simulink model "StateSpace"  (R2022a)
settings: Solver=ode113  StartTime=0.0  StopTime=10  MaxStep=1e-3  RelTol=1e-6
undefined symbols (not defined in the file): k
settings Model: Creator=Administrator  LastModifiedBy=Administrator
settings SolverCC: NumberNewtonIterations=100  MaxConsecutiveMinStep=10  SolverJacobianMethodControl=FullAnalytical  DaesscMode=FullDebug  ShapePreserveControl=EnableAll  ZeroCrossAlgorithm=Adaptive  SolverResetMethod=Robust  ODENIntegrationMethod=ode14x

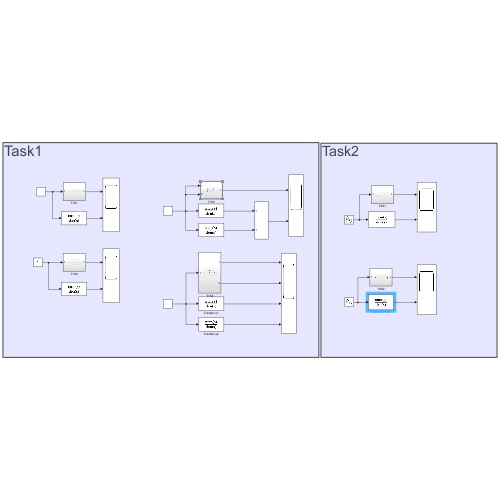
[thumbnail: Simulink's stored preview of the top-level diagram]
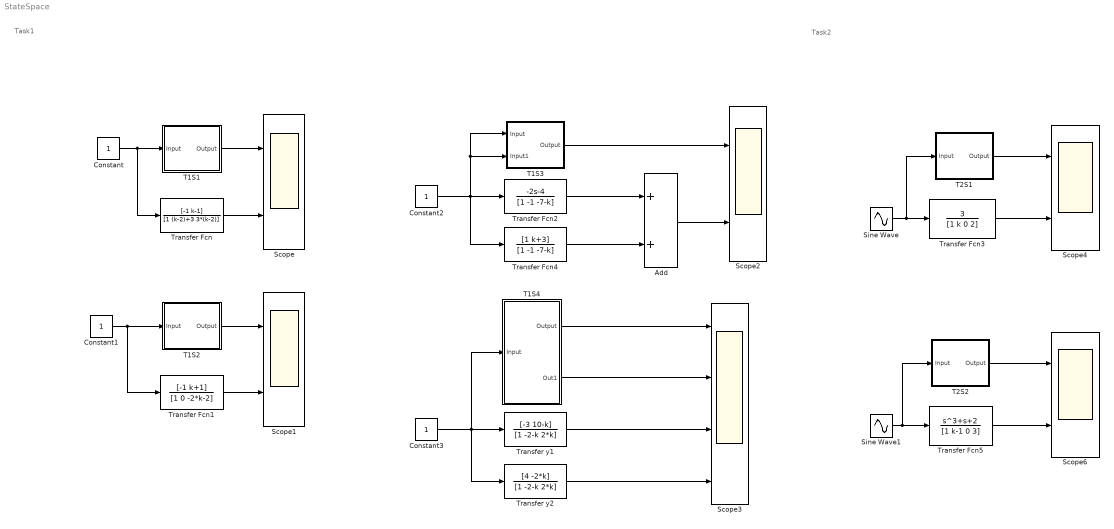
== system StateSpace ==
  note: Task2
  note: Task1
  Add : Sum  RndMeth=Nearest
  Constant{,1..3} (4 alike) : Constant
  Scope{,1..2,4,6} (5 alike) : Scope  NumInputPorts=2
  Scope3 : Scope  NumInputPorts=4
  Sine Wave : Sin  Amplitude=3  Frequency=2  SampleTime=0
  Sine Wave1 : Sin  Amplitude=3  Frequency=2  SampleTime=0
  T1S1 : Subsystem
  T1S2 : Subsystem
  T1S3 : Subsystem
  T1S4 : Subsystem
  T2S1 : Subsystem
  T2S2 : Subsystem
  Transfer Fcn : TransferFcn  Numerator=[-1 k-1]  Denominator=[1 (k-2)+3 3*(k-2)]
  Transfer Fcn1 : TransferFcn  Numerator=[-1 k+1]  Denominator=[1 0 -2*k-2]
  Transfer Fcn2 : TransferFcn  Numerator=[-2 -4]  Denominator=[1 -1 -7-k]
  Transfer Fcn3 : TransferFcn  Numerator=[3]  Denominator=[1 k 0 2]
  Transfer Fcn4 : TransferFcn  Numerator=[1 k+3]  Denominator=[1 -1 -7-k]
  Transfer Fcn5 : TransferFcn  Numerator=[1 0 1 2]  Denominator=[1 k-1 0 3]
  Transfer y1 : TransferFcn  Numerator=[-3 10-k]  Denominator=[1 -2-k 2*k]
  Transfer y2 : TransferFcn  Numerator=[4 -2*k]  Denominator=[1 -2-k 2*k]
  wires:
  Constant/1 -> Transfer Fcn/1, T1S1/1(Input)
  T1S1/1(Output) -> Scope/1
  Transfer Fcn/1 -> Scope/2
  Constant1/1 -> Transfer Fcn1/1, T1S2/1(Input)
  Transfer Fcn1/1 -> Scope1/2
  T1S2/1(Output) -> Scope1/1
  T1S3/1(Output) -> Scope2/1
  Transfer Fcn2/1 -> Add/1
  Constant2/1 -> T1S3/1(Input), T1S3/2(Input1), Transfer Fcn4/1, Transfer Fcn2/1
  Constant3/1 -> T1S4/1(Input), Transfer y2/1, Transfer y1/1
  Transfer y1/1 -> Scope3/3
  T1S4/1(Output) -> Scope3/1
  Add/1 -> Scope2/2
  Transfer Fcn4/1 -> Add/2
  T1S4/2(Out1) -> Scope3/2
  Transfer y2/1 -> Scope3/4
  Sine Wave/1 -> Transfer Fcn3/1, T2S1/1(Input)
  Transfer Fcn3/1 -> Scope4/2
  Sine Wave1/1 -> T2S2/1(Input), Transfer Fcn5/1
  Transfer Fcn5/1 -> Scope6/2
  T2S1/1(Output) -> Scope4/1
  T2S2/1(Output) -> Scope6/1

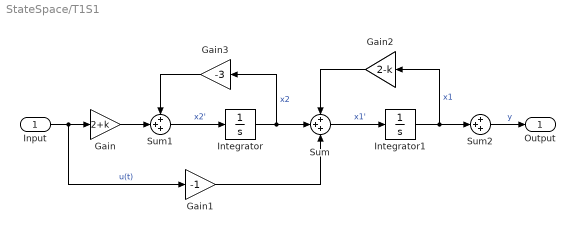
== system StateSpace/T1S1 ==
  Input : Inport
  Gain : Gain  Gain=2+k
  Gain1 : Gain  Gain=-1
  Gain2 : Gain  Gain=2-k
  Gain3 : Gain  Gain=-3
  Integrator : Integrator
  Integrator1 : Integrator
  Sum : Sum  Inputs=+++
  Sum1 : Sum  Inputs=+++
  Sum2 : Sum  Inputs=+++
  Output : Outport
  wires:
  Gain2/1 -> Sum/1
  Sum/1 -> Integrator1/1  "x1'"
  Integrator1/1 -> Sum2/2, Gain2/1  "x1"
  Input/1 -> Gain1/1, Gain/1  "u(t)"
  Gain/1 -> Sum1/2
  Sum1/1 -> Integrator/1  "x2'"
  Integrator/1 -> Gain3/1, Sum/2  "x2"
  Gain1/1 -> Sum/3
  Sum2/1 -> Output/1  "y"
  Gain3/1 -> Sum1/1

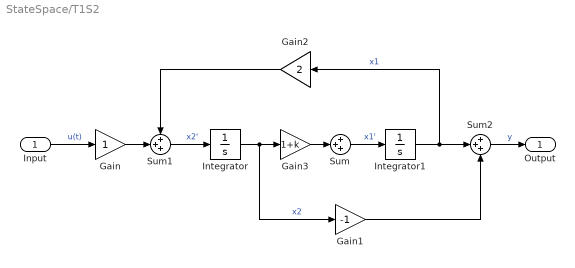
== system StateSpace/T1S2 ==
  Input : Inport
  Gain : Gain
  Gain1 : Gain  Gain=-1
  Gain2 : Gain  Gain=2
  Gain3 : Gain  Gain=1+k
  Integrator : Integrator
  Integrator1 : Integrator
  Sum : Sum  Inputs=+++
  Sum1 : Sum  Inputs=+++
  Sum2 : Sum  Inputs=+++
  Output : Outport
  wires:
  Gain2/1 -> Sum1/1
  Sum/1 -> Integrator1/1  "x1'"
  Integrator1/1 -> Sum2/2, Gain2/1  "x1"
  Input/1 -> Gain/1  "u(t)"
  Gain/1 -> Sum1/2
  Sum1/1 -> Integrator/1  "x2'"
  Integrator/1 -> Gain1/1, Gain3/1  "x2"
  Sum2/1 -> Output/1  "y"
  Gain3/1 -> Sum/2
  Gain1/1 -> Sum2/3

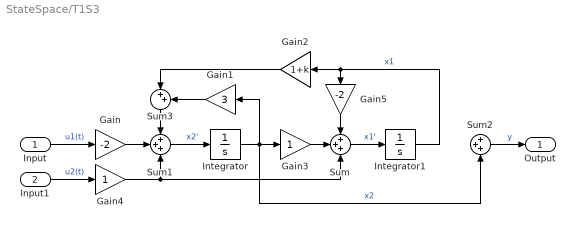
== system StateSpace/T1S3 ==
  Input : Inport
  Input1 : Inport  Port=2
  Gain : Gain  Gain=-2
  Gain1 : Gain  Gain=3
  Gain2 : Gain  Gain=1+k
  Gain3 : Gain
  Gain4 : Gain
  Gain5 : Gain  Gain=-2
  Integrator : Integrator
  Integrator1 : Integrator
  Sum : Sum  Inputs=+++
  Sum1 : Sum  Inputs=+++
  Sum2 : Sum  Inputs=+++
  Sum3 : Sum  Inputs=|++
  Output : Outport
  wires:
  Gain2/1 -> Sum3/1
  Sum/1 -> Integrator1/1  "x1'"
  Integrator1/1 -> Gain2/1, Gain5/1  "x1"
  Input/1 -> Gain/1  "u1(t)"
  Gain/1 -> Sum1/2
  Sum1/1 -> Integrator/1  "x2'"
  Integrator/1 -> Sum2/3, Gain1/1, Gain3/1  "x2"
  Sum2/1 -> Output/1  "y"
  Gain3/1 -> Sum/2
  Input1/1 -> Gain4/1  "u2(t)"
  Gain4/1 -> Sum/3, Sum1/3
  Sum3/1 -> Sum1/1
  Gain1/1 -> Sum3/2
  Gain5/1 -> Sum/1

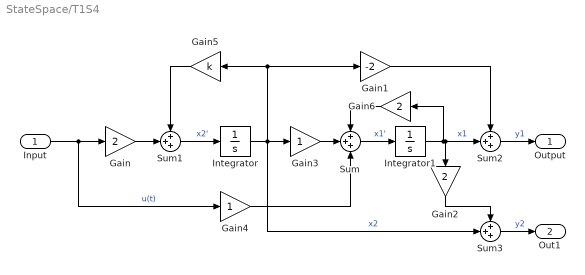
== system StateSpace/T1S4 ==
  Input : Inport
  Gain : Gain  Gain=2
  Gain1 : Gain  Gain=-2
  Gain2 : Gain  Gain=2
  Gain3 : Gain
  Gain4 : Gain
  Gain5 : Gain  Gain=k
  Gain6 : Gain  Gain=2
  Integrator : Integrator
  Integrator1 : Integrator
  Sum{,1..3} (4 alike) : Sum  Inputs=+++
  Output : Outport
  Out1 : Outport  Port=2
  wires:
  Sum/1 -> Integrator1/1  "x1'"
  Integrator1/1 -> Gain6/1, Sum2/2, Gain2/1  "x1"
  Input/1 -> Gain4/1, Gain/1  "u(t)"
  Gain/1 -> Sum1/2
  Sum1/1 -> Integrator/1  "x2'"
  Integrator/1 -> Gain3/1, Gain1/1, Gain5/1, Sum3/2  "x2"
  Sum2/1 -> Output/1  "y1"
  Gain3/1 -> Sum/2
  Sum3/1 -> Out1/1  "y2"
  Gain1/1 -> Sum2/1
  Gain2/1 -> Sum3/1
  Gain4/1 -> Sum/3
  Gain5/1 -> Sum1/1
  Gain6/1 -> Sum/1

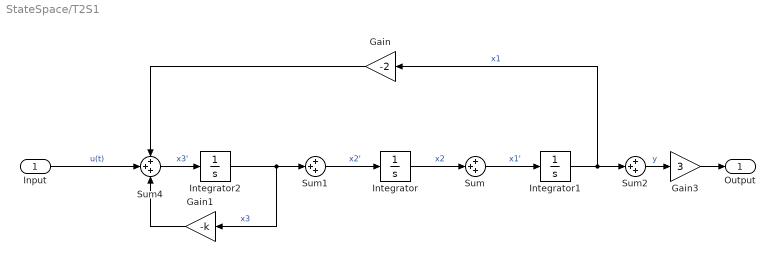
== system StateSpace/T2S1 ==
  Input : Inport
  Gain : Gain  Gain=-2
  Gain1 : Gain  Gain=-k
  Gain3 : Gain  Gain=3
  Integrator : Integrator
  Integrator1 : Integrator
  Integrator2 : Integrator
  Sum{,1..2,4} (4 alike) : Sum  Inputs=+++
  Output : Outport
  wires:
  Sum/1 -> Integrator1/1  "x1'"
  Integrator1/1 -> Gain/1, Sum2/2  "x1"
  Sum1/1 -> Integrator/1  "x2'"
  Integrator/1 -> Sum/2  "x2"
  Sum2/1 -> Gain3/1  "y"
  Integrator2/1 -> Sum1/2, Gain1/1  "x3"
  Gain3/1 -> Output/1
  Gain/1 -> Sum4/1
  Sum4/1 -> Integrator2/1  "x3'"
  Input/1 -> Sum4/2  "u(t)"
  Gain1/1 -> Sum4/3

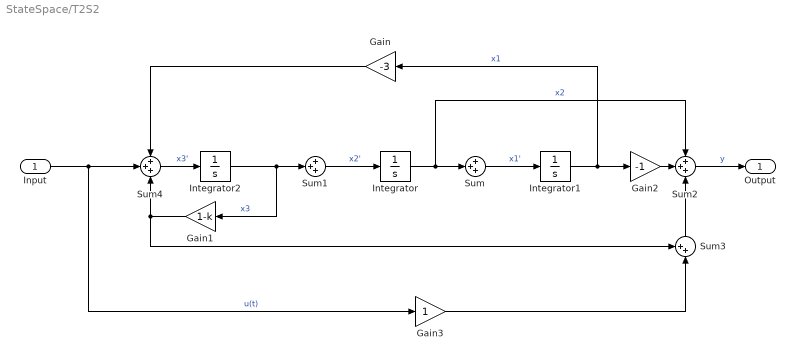
== system StateSpace/T2S2 ==
  Input : Inport
  Gain : Gain  Gain=-3
  Gain1 : Gain  Gain=1-k
  Gain2 : Gain  Gain=-1
  Gain3 : Gain
  Integrator : Integrator
  Integrator1 : Integrator
  Integrator2 : Integrator
  Sum{,1..2,4} (4 alike) : Sum  Inputs=+++
  Sum3 : Sum  Inputs=++|
  Output : Outport
  wires:
  Sum/1 -> Integrator1/1  "x1'"
  Integrator1/1 -> Gain2/1, Gain/1  "x1"
  Sum1/1 -> Integrator/1  "x2'"
  Integrator/1 -> Sum2/1, Sum/2  "x2"
  Sum2/1 -> Output/1  "y"
  Integrator2/1 -> Sum1/2, Gain1/1  "x3"
  Gain/1 -> Sum4/1
  Sum4/1 -> Integrator2/1  "x3'"
  Input/1 -> Gain3/1, Sum4/2  "u(t)"
  Gain1/1 -> Sum3/1, Sum4/3
  Sum3/1 -> Sum2/3
  Gain2/1 -> Sum2/2
  Gain3/1 -> Sum3/2
